simulink model "test1"  (R2025a)
settings: Solver=ode23tb  StartTime=0.0  StopTime=5  RelTol=1e-3
model workspace (MAT data in the model file):
  kd = 0.15
  m = 5
  mw = 2.5
settings Model: Creator=wzy  LastModifiedBy=wzy

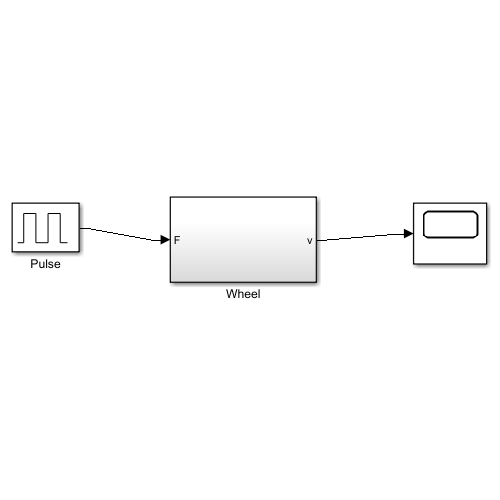
[thumbnail: Simulink's stored preview of the top-level diagram]
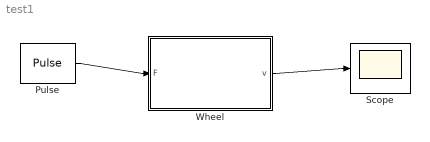
== system test1 ==
  Pulse : DiscretePulseGenerator  PulseType=Time based  Amplitude=2  Period=20  PulseWidth=15
  Scope : Scope
  Wheel : Subsystem
  wires:
  Pulse/1 -> Wheel/1(F)
  Wheel/1(v) -> Scope/1

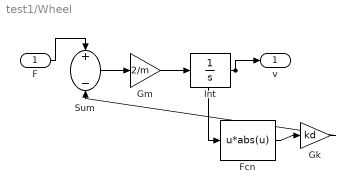
== system test1/Wheel ==
  F : Inport
  Fcn : Fcn  Expr=u*abs(u)
  Gk : Gain  Gain=kd
  Gm : Gain  Gain=2/m
  Int : Integrator
  Sum : Sum  Inputs=+-
  v : Outport
  wires:
  F/1 -> Sum/1
  Sum/1 -> Gm/1
  Gm/1 -> Int/1
  Int/1 -> v/1, Fcn/1
  Fcn/1 -> Gk/1
  Gk/1 -> Sum/2
